simulink model "eBikeFinal"  (R2020b)
settings: Solver=daessc  StartTime=0.0  StopTime=60  FixedStep=1/500  AbsTol=1e-3  EnableMultiTasking=on
PreLoadFcn:
  | xh = 2*pi/60*[0:10:200];     % rpm to rad/s
  | yh = 50*(1-exp(-(max(xh)-xh)/2));
  | load bicycle_params
undefined symbols (not defined in the file or in its folder): sigbuilder_block
libraries: fl_lib x24, nesl_utility x15, sdl_lib x12, simulink x4, clutch_lib x3, motor_lib x3, LinearBrake_lib x2, pid_lib x2
settings Model: Creator=emcgarri  LastModifiedBy=amyyang
settings DataIOCC: SaveFormat=Array
settings OptimizationCC: BlockReduction=off  BufferReuse=off  LifeSpan=inf
settings DebuggingCC: ReadBeforeWriteMsg=DisableAll  WriteAfterWriteMsg=DisableAll  WriteAfterReadMsg=DisableAll  AlgebraicLoopMsg=none  UnderspecifiedInitializationDetection=Classic  MergeDetectMultiDrivingBlocksExec=none  MultiTaskDSMMsg=none  UnconnectedInputMsg=none  UnconnectedOutputMsg=none  UnconnectedLineMsg=none  SFUnexpectedBacktrackingDiag=warning  SFNoUnconditionalDefaultTransitionDiag=warning  SFExecutionAtInitializationDiag=none  ArithmeticOperatorsInVariantConditions=warning
settings HardwareCC: ProdBitPerPointer=32  ProdBitPerSizeT=32  ProdBitPerPtrDiffT=32  ProdLargestAtomicFloat=None  ProdIntDivRoundTo=Undefined  ProdEndianess=Unspecified  ProdWordSize=32  ProdHWDeviceType=32-bit Generic
settings ModelReferenceCC: UpdateModelReferenceTargets=IfOutOfDate  PropagateSignalLabelsOutOfModel=off
settings SFSimCC: SFSimEcho=off  SimUseLocalCustomCode=off
settings RTWCC: RTWUseLocalCustomCode=off
settings CodeAppCC: StateflowObjectComments=on
settings GRTTargetCC: TargetLangStandard=C89/C90 (ANSI)
settings ConfigComp: CovMetricSettings=dw  CovSaveCumulativeToWorkspaceVar=on  CovSaveSingleToWorkspaceVar=on  CovExternalEMLEnable=off  CovSFcnEnable=off
settings SimscapeCC: SimscapeNormalizeSystem=off

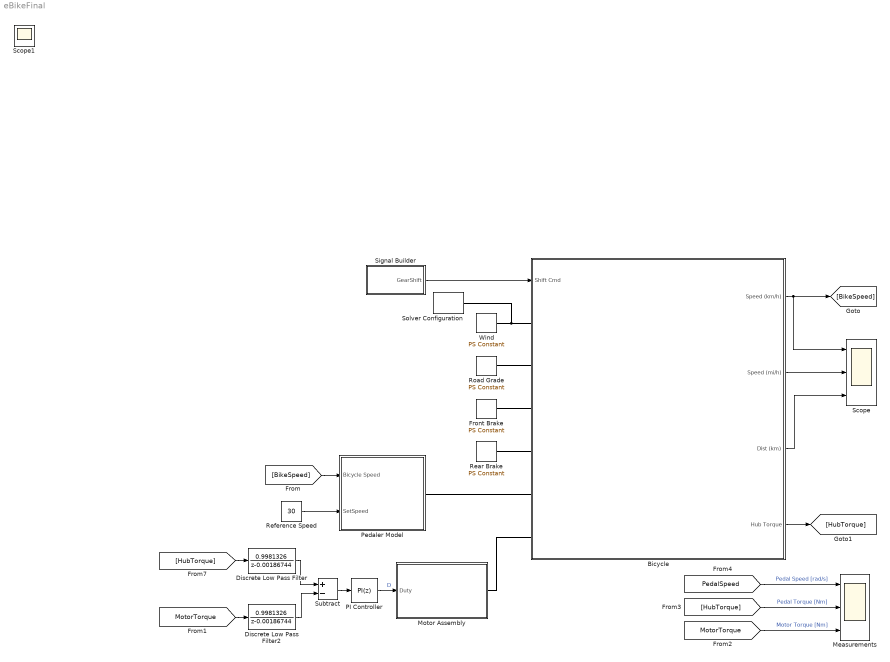
== system eBikeFinal ==
  Bicycle : Subsystem
      mask Display:
      | image(imread('FullBike.png'));
      | color('Orange')
      | port_label('input', 1, 'Gear');
      | port_label('lconn', 1, 'W');
      | port_label('lconn', 2, 'T');
      | port_label('lconn', 3, 'FB');
      | port_label('lconn', 4, 'RB');
      | port_label('lconn', 5, 'C');
      | port_label('lconn', 6, 'FH');
      | port_label('output', 1, 'Spd1');
      | port_label('output', 2, 'Spd2');
      | port_label('output', 3, 'Dist');
      | port_label('output', 4, 'TH');
  Discrete Low Pass Filter : DiscreteTransferFcn  Numerator=[0.9981326]  Denominator=[1 -0.00186744]  SampleTime=0.05
  Discrete Low Pass Filter2 : DiscreteTransferFcn  Numerator=[0.9981326]  Denominator=[1 -0.00186744]  SampleTime=0.05
  Front Brake : fl_lib/Physical Signals/Sources/PS Constant  constant=0 N
  Measurements : Scope  NumInputPorts=3
  Motor Assembly : Subsystem
      mask Display:
      | image(imread('MotorAssembly.png'));
      | color('Red');
      | port_label('input', 1, 'Duty');
      | port_label('rconn', 1, 'T');
  PI Controller : pid_lib/PID Controller  Controller=PI  Form=Parallel  TimeDomain=Discrete-time  UseExternalTs=off  SampleTime=0.05  IntegratorMethod=Forward Euler  FilterMethod=Forward Euler  ControllerParametersSource=internal  P=0.005  I=0.01  D=0.05  UseFilter=on  N=100  TunerSelectOption=Transfer Function Based (PID Tuner App)  InitialConditionSource=internal  InitialConditionForIntegrator=0  InitialConditionForFilter=0  DifferentiatorICPrevScaledInput=0  ExternalReset=none  IgnoreLimit=on  TrackingMode=off  Kt=1  LimitOutput=on  SatLimitsSource=internal  UpperSaturationLimit=1  LowerSaturationLimit=0  LinearizeAsGain=off  AntiWindupMode=clamping  Kb=1  POutMin=[]  POutMax=[]  IOutMin=[]  IOutMax=[]  DOutMin=[]  DOutMax=[]  NOutMin=[]  NOutMax=[]  SumOutMin=[]  SumOutMax=[]  SaturationOutMin=[]  SaturationOutMax=[]  PParamMin=[]  PParamMax=[]  IParamMin=[]  IParamMax=[]  DParamMin=[]  DParamMax=[]  NParamMin=[]  NParamMax=[]  KbParamMin=[]  KbParamMax=[]  KtParamMin=[]  KtParamMax=[]  KbOutMin=[]  KbOutMax=[]  KtOutMin=[]  KtOutMax=[]  IntegratorOutMin=[]  IntegratorOutMax=[]  FilterOutMin=[]  FilterOutMax=[]  SumI1OutMin=[]  SumI1OutMax=[]  SumI2OutMin=[]  SumI2OutMax=[]  SumI3OutMin=[]  SumI3OutMax=[]  SumI4OutMin=[]  SumI4OutMax=[]  SumDOutMin=[]  SumDOutMax=[]  DifferentiatorOutMin=[]  DifferentiatorOutMax=[]  FilterDiffOutCoefMin=[]  FilterDiffOutCoefMax=[]  ReciprocalOutMin=[]  ReciprocalOutMax=[]  SumDenOutMin=[]  SumDenOutMax=[]  SumNumOutMin=[]  SumNumOutMax=[]  DivideOutMin=[]  DivideOutMax=[]  UdiffTsProdOutMin=[]  UdiffTsProdOutMax=[]  NTsProdOutMin=[]  NTsProdOutMax=[]  UintegralTsProdOutMin=[]  UintegralTsProdOutMax=[]  UngainTsProdOutMin=[]  UngainTsProdOutMax=[]  IntegratorContinuousStateAttributes=''  IntegratorStateMustResolveToSignalObject=off  IntegratorRTWStateStorageClass=Auto  FilterContinuousStateAttributes=''  FilterStateMustResolveToSignalObject=off  FilterRTWStateStorageClass=Auto  ParallelPVariant=InternalParameters  IdealPVariant=Disabled  IVariant=InternalParameters  DVariant=Disabled  IntegratorVariant=Discrete  SatVariant=Enabled  AWVariant=DiscClampingParallel  PCopyVariant=Disabled  TRVariant=Disabled  FdbkBlocksVariant=Forward  IdealPFdbkVariant=Disabled  SatFdbkVariant=Disabled  DerivativeFilterVariant=Disabled  NVariant=Disabled  NCopyVariant=Disabled_SignalSpec  FilterICVariant=Disabled  IntegratorICVariant=InternalICs  ExternalResetVariant=Disabled  TRSumVariant=Passthrough  SumFdbkVariant=Disabled  SumVariant=Sum_PI  TsampFilterVariant=InternalTs  TsampNgainVariant=Passthrough  TsampIntegralVariant=Passthrough  ExternalSaturationOutDataTypeStr=Inherit: Same as second input
  Pedaler Model : Subsystem
      mask Display: image(imread('RiderIcon.png'));
  Rear Brake : fl_lib/Physical Signals/Sources/PS Constant  constant=0 N
  Reference Speed : Constant  Value=30
  Road Grade : fl_lib/Physical Signals/Sources/PS Constant  constant=0 deg
  Scope : Scope  NumInputPorts=3
  Signal Builder : Subsystem  Tag=STV Subsys  LoadFcn=sigbuilder_block('load');  StartFcn=sigbuilder_block('start');  StopFcn=sigbuilder_block('stop');  ClipboardFcn=sigbuilder_block('clipboard');  mask(Sigbuilder block){tuvar=[0:10]}
      mask help: Simulink:masks:SigbuilderBlock_MD
      mask init:
      | if ~strcmp(get_param(bdroot(gcbh),'SimulationStatus'),'stopped') tuvar = sigbuilder_block('maskInit'); end
      settings: CopyFcn=sigbuilder_block('copy');  DeleteFcn=sigbuilder_block('delete');  ModelCloseFcn=sigbuilder_block('modelClose');  PreSaveFcn=sigbuilder_block('preSave');  PauseFcn=sigbuilder_block('pause');  ContinueFcn=sigbuilder_block('continue');  NameChangeFcn=sigbuilder_block('namechange');  OpenFcn=sigbuilder_block('open',[306 225.6 549.6 399.6 ]);  CloseFcn=sigbuilder_block('close');
      mask Display: plot(0, 0, 100, 100,[2, 2, 32, 32, 2], [68, 8, 8, 68, 68],[32, 2], [38, 38], [32, 19, 2],[53, 60, 44], [32, 17, 17, 2],[16, 16, 31, 31]);txt = getActiveGroup(gcbh);text(2, 100, txt,'verticalAlignment', 'top');
  Solver Configuration : nesl_utility/Solver Configuration  PhysicalDomain=network_engine_domain  SubClassName=solver  LeftPortType=input  RightPortType=generic  Tones=[]  Harmonics=[]  SimulateNoise=off  Profile=off  UseLocalSampling=off  EnableSwitchedLinearOptims=on  FrequencyDomain=off  UseCCode=off  RelTol=0.001  AbsTol=1e-06  MinStep=1e-09  ToWorkspace=off  RevertToSquareIcSolve=off  NumHomotopyIterations=100  PhasorMode=off  PhasorModeNumHarmonics=1  DoDC=off  ResidualTolerance=1e-09  UseLocalSolver=off  LocalSolverChoice=NE_BACKWARD_EULER_ADVANCER  LocalSolverSampleTime=1e-3  DoFixedCost=off  MaxNonlinIter=3  MaxModeIter=2  ComputeImpulses=off  ImpulseIterations=1  LinearAlgebra=Sparse  EquationFormulation=NE_TIME_EF  DelaysMemoryBudget=1024  AutomaticFiltering=off  FilteringTimeConstant=0.001  PartitionStorageMethod=AS_NEEDED  PartitionMemoryBudget=1024  PartitionMethod=FAST
  Subtract : Sum  Inputs=+-
  Wind : fl_lib/Physical Signals/Sources/PS Constant  constant=0 m/s
  Scope1 : Scope
  wires:
  [BikeSpeed] -> Pedaler Model/1(Bicycle Speed)
  Reference Speed/1 -> Pedaler Model/2(SetSpeed)
  [HubTorque] -> Measurements/2  "Pedal Torque [Nm]"
  [MotorTorque] -> Measurements/3  "Motor Torque [Nm]"
  [PedalSpeed] -> Measurements/1  "Pedal Speed [rad/s]"
  Signal Builder/1(GearShift) -> Bicycle/1(Shift Cmd)
  PI Controller/1 -> Motor Assembly/1(Duty)  "D"
  [MotorTorque] -> Discrete Low Pass Filter2/1
  Subtract/1 -> PI Controller/1
  [HubTorque] -> Discrete Low Pass Filter/1
  Discrete Low Pass Filter2/1 -> Subtract/2
  Discrete Low Pass Filter/1 -> Subtract/1
  Bicycle/2(Speed (mi/h)) -> Scope/2
  Bicycle/3(Dist (km)) -> Scope/3
  Bicycle/4(Hub Torque) -> [HubTorque]
  Bicycle/1(Speed (km/h)) -> Scope/1, [BikeSpeed]
  connections:
  Bicycle/LConn5 -- Pedaler Model/RConn1
  Bicycle/LConn3 -- Front Brake/RConn1
  Bicycle/LConn4 -- Rear Brake/RConn1
  Bicycle/LConn2 -- Road Grade/RConn1
  Wind/RConn1 -- Bicycle/LConn1 -- Solver Configuration/RConn1
  Bicycle/LConn6 -- Motor Assembly/RConn1

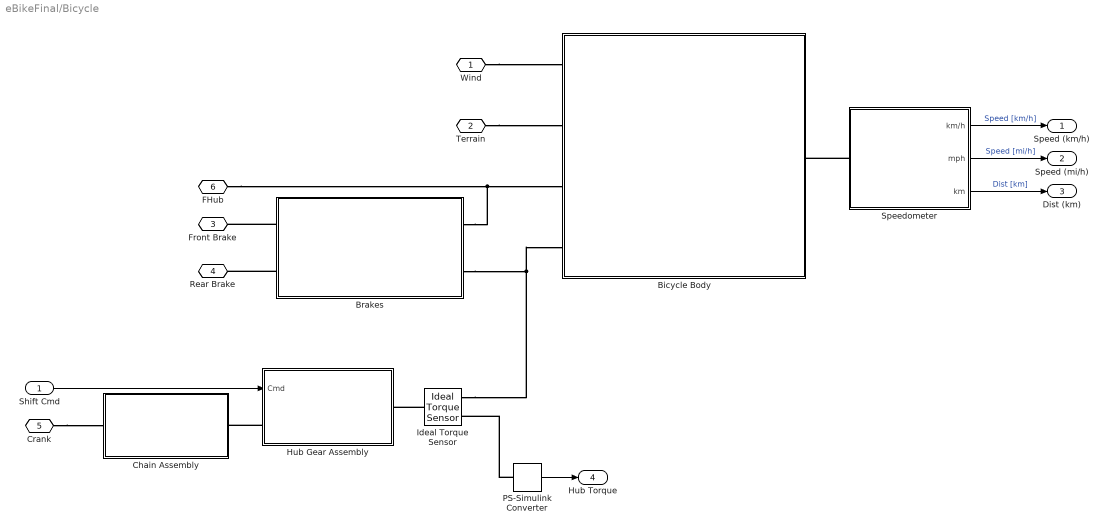
== system eBikeFinal/Bicycle ==
  Shift Cmd : Inport
  "Bicycle Body " : Subsystem  mask(Vehicle){rider_mass=80, rider_area=0.8, drag_coeff=0.5, bike_mass=13, front_axle=47, rear_axle=65, CG_height=120, rim_radius=311, tire_height=41, tire_friction_s=1.0, tire_friction_k=0.7, roll_resist=0.004}
      mask prompts: rider_mass "Mass [kg]"; rider_area "Area [m^2]"; drag_coeff "Drag Coefficient"; bike_mass "Frame Mass [kg]"; front_axle "Front Axle Loc [cm]"; rear_axle "Real Axle Loc [cm]"; CG_height "CG Height [cm]"; rim_radius "Rim Radius [mm]"; tire_height "Tire Height [mm]"; tire_friction_s "Static Tire Friction"; tire_friction_k "Kinetic Tire Friction"; roll_resist "Rolling Resistance"
      mask help:
      | This block represents a simple bicycle body with drive attachments on both
      | the front and rear hubs.
      mask Display:
      | image(imread('BikeIcon.png'));
      | color('Orange')
      | port_label('lconn', 1, 'W');
      | port_label('lconn', 2, 'T');
      | port_label('rconn', 1, 'H');
      | port_label('lconn', 3, 'F');
      | port_label('lconn', 4, 'R');
  Brakes : Subsystem
      mask Display:
      | image(imread('HandleBars.png'));
      | color('Red');
      | port_label('lconn', 1, 'FCmd');
      | port_label('lconn', 2, 'RCmd');
      | port_label('rconn', 1, 'FB');
      | port_label('rconn', 2, 'RB');
  Chain Assembly : Subsystem
      mask Display:
      | image(imread('ChainDrive.png'))
      | color('Orange')
      | port_label('lconn', 1, 'C');
      | port_label('rconn', 1, 'H');
  Hub Gear Assembly : Subsystem
      mask Display:
      | image(imread('HubTrans.png'))
      | color('Orange')
      | port_label('input', 1, 'Cmd');
      | port_label('lconn', 1, 'A');
      | port_label('rconn', 1, 'H');
  Ideal Torque Sensor : fl_lib/Mechanical/Mechanical Sensors/Ideal Torque Sensor
  PS-Simulink Converter : nesl_utility/PS-Simulink Converter  PhysicalDomain=network_engine_domain  SubClassName=ps_output  LeftPortType=input  RightPortType=output  PseudoPeriodic=off  Frequencies=[]  Unit=N*m  AffineConversion=off
  Speedometer : Subsystem  mask(Speedometer){}
      mask help:
      | Simple speedometer/odometer. The input signal should be a physical signal
      | with units of m/s. The output signals are km/h, mi/h and km traveled as
      | Simulink signals for convenient plotting.
      mask Display:
      | image(imread('SpeedometerIcon.png'));
      | color('Orange')
      | port_label('lconn', 1, 'H');
      | port_label('output', 1, 'km/h');
      | port_label('output', 2, 'mi/h');
      | port_label('output', 3, 'km');
  Wind : PMIOPort  Side=Left
  Terrain : PMIOPort  Port=2  Side=Left
  Front Brake : PMIOPort  Port=3  Side=Left
  Rear Brake : PMIOPort  Port=4  Side=Left
  Crank : PMIOPort  Port=5  Side=Left
  FHub : PMIOPort  Port=6  Side=Left
  Speed (km/h) : Outport  VectorParamsAs1DForOutWhenUnconnected=off
  Speed (mi/h) : Outport  Port=2  VectorParamsAs1DForOutWhenUnconnected=off
  Dist (km) : Outport  Port=3  VectorParamsAs1DForOutWhenUnconnected=off
  Hub Torque : Outport  Port=4  VectorParamsAs1DForOutWhenUnconnected=off
  wires:
  Speedometer/1(km/h) -> Speed (km/h)/1  "Speed [km/h]"
  Speedometer/2(mph) -> Speed (mi/h)/1  "Speed [mi/h]"
  Speedometer/3(km) -> Dist (km)/1  "Dist [km]"
  Shift Cmd/1 -> Hub Gear Assembly/1(Cmd)
  PS-Simulink Converter/1 -> Hub Torque/1
  connections:
  Wind/RConn1 -- "Bicycle Body "/LConn1
  Terrain/RConn1 -- "Bicycle Body "/LConn2
  Speedometer/LConn1 -- "Bicycle Body "/RConn1
  Brakes/LConn1 -- Front Brake/RConn1
  Brakes/LConn2 -- Rear Brake/RConn1
  Hub Gear Assembly/LConn1 -- Chain Assembly/RConn1
  FHub/RConn1 -- Brakes/RConn1 -- "Bicycle Body "/LConn3
  Brakes/RConn2 -- "Bicycle Body "/LConn4 -- Ideal Torque Sensor/RConn1
  Crank/RConn1 -- Chain Assembly/LConn1
  PS-Simulink Converter/LConn1 -- Ideal Torque Sensor/RConn2
  Ideal Torque Sensor/LConn1 -- Hub Gear Assembly/RConn1

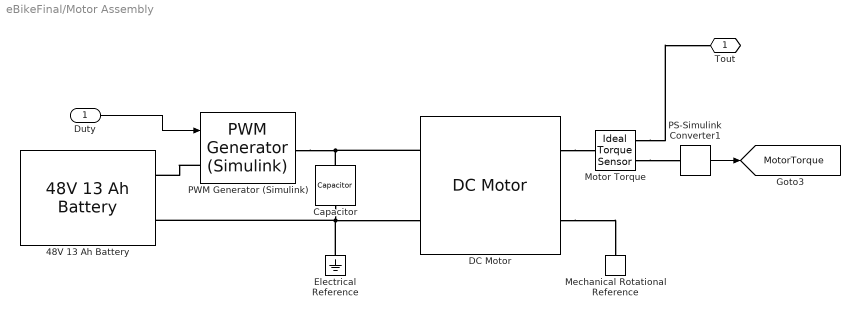
== system eBikeFinal/Motor Assembly ==
  Duty : Inport
  48V 13 Ah Battery : motor_lib/48V 13 Ah Battery  SystemSampleTime=-1  VariantActivationTime=update diagram  Latency=0  AutoFrameSizeCalculation=off
  Capacitor : fl_lib/Electrical/Electrical Elements/Capacitor  c=0.2 F  r=1e-6 Ohm  g=0 1/Ohm  i_specify=off  i_priority=None  i=0 A  i_nominal_specify=off  i_nominal_unit=A  i_nominal_value=1  v_specify=off  v_priority=None  v=0 V  v_nominal_specify=off  v_nominal_unit=V  v_nominal_value=1  vc_specify=on  vc_priority=High  vc=0 V  vc_nominal_specify=off  vc_nominal_unit=V  vc_nominal_value=1
  DC Motor : motor_lib/DC Motor  SystemSampleTime=-1  VariantActivationTime=update diagram  Latency=0  AutoFrameSizeCalculation=off
  Electrical Reference : fl_lib/Electrical/Electrical Elements/Electrical Reference
  Mechanical Rotational Reference : fl_lib/Mechanical/Rotational Elements/Mechanical Rotational Reference
  Motor Torque : fl_lib/Mechanical/Mechanical Sensors/Ideal Torque Sensor
  PS-Simulink Converter1 : nesl_utility/PS-Simulink Converter  PhysicalDomain=network_engine_domain  SubClassName=ps_output  LeftPortType=input  RightPortType=output  PseudoPeriodic=off  Frequencies=[]  Unit=1  AffineConversion=off
  PWM Generator (Simulink) : motor_lib/PWM Generator  (Simulink)  freq=50  Ts=2e-4
  Tout : PMIOPort  Side=Right
  tag scope: MotorTorque=global
  wires:
  PS-Simulink Converter1/1 -> [MotorTorque]
  Duty/1 -> PWM Generator (Simulink)/1
  connections:
  DC Motor/RConn2 -- Mechanical Rotational Reference/LConn1
  DC Motor/LConn1 -- PWM Generator (Simulink)/RConn1 -- Capacitor/LConn1
  PWM Generator (Simulink)/LConn1 -- 48V 13 Ah Battery/RConn1
  DC Motor/RConn1 -- Motor Torque/LConn1
  Motor Torque/RConn2 -- PS-Simulink Converter1/LConn1
  Motor Torque/RConn1 -- Tout/RConn1
  Capacitor/RConn1 -- Electrical Reference/LConn1 -- 48V 13 Ah Battery/RConn2 -- DC Motor/LConn2

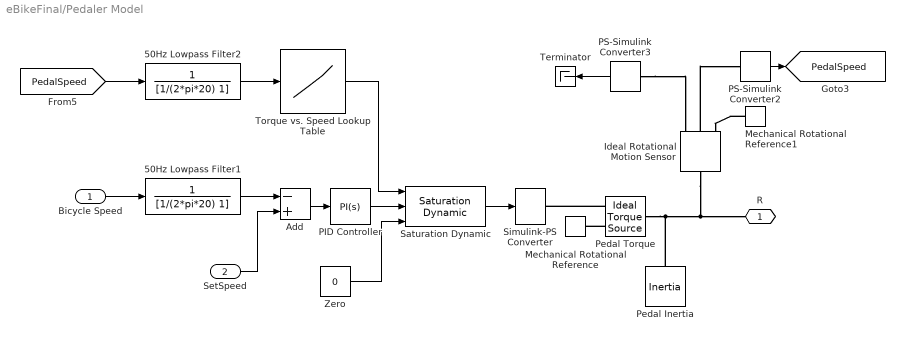
== system eBikeFinal/Pedaler Model ==
  Bicycle Speed : Inport
  SetSpeed : Inport  Port=2
  50Hz Lowpass Filter1 : TransferFcn  Denominator=[1/(2*pi*20) 1]
  50Hz Lowpass Filter2 : TransferFcn  Denominator=[1/(2*pi*20) 1]
  Add : Sum  Inputs=-+
  Ideal Rotational Motion Sensor : fl_lib/Mechanical/Mechanical Sensors/Ideal Rotational Motion Sensor  wrap_angle=simscape.enum.onoff.off  offset=0 rad
  Mechanical Rotational Reference : fl_lib/Mechanical/Rotational Elements/Mechanical Rotational Reference
  Mechanical Rotational Reference1 : fl_lib/Mechanical/Rotational Elements/Mechanical Rotational Reference
  PID Controller : pid_lib/PID Controller  Controller=PI  Form=Parallel  TimeDomain=Continuous-time  UseExternalTs=off  SampleTime=-1  IntegratorMethod=Forward Euler  FilterMethod=Forward Euler  ControllerParametersSource=internal  P=20  I=0  D=0  UseFilter=on  N=100  TunerSelectOption=Transfer Function Based (PID Tuner App)  InitialConditionSource=internal  InitialConditionForIntegrator=0  InitialConditionForFilter=0  DifferentiatorICPrevScaledInput=0  ExternalReset=none  TrackingMode=off  Kt=1  LimitOutput=off  SatLimitsSource=internal  UpperSaturationLimit=50  LowerSaturationLimit=0  LinearizeAsGain=on  AntiWindupMode=clamping  Kb=1  POutMin=[]  POutMax=[]  IOutMin=[]  IOutMax=[]  DOutMin=[]  DOutMax=[]  NOutMin=[]  NOutMax=[]  SumOutMin=[]  SumOutMax=[]  SaturationOutMin=[]  SaturationOutMax=[]  PParamMin=[]  PParamMax=[]  IParamMin=[]  IParamMax=[]  DParamMin=[]  DParamMax=[]  NParamMin=[]  NParamMax=[]  KbParamMin=[]  KbParamMax=[]  KtParamMin=[]  KtParamMax=[]  KbOutMin=[]  KbOutMax=[]  KtOutMin=[]  KtOutMax=[]  IntegratorOutMin=[]  IntegratorOutMax=[]  FilterOutMin=[]  FilterOutMax=[]  SumI1OutMin=[]  SumI1OutMax=[]  SumI2OutMin=[]  SumI2OutMax=[]  SumI3OutMin=[]  SumI3OutMax=[]  SumI4OutMin=[]  SumI4OutMax=[]  SumDOutMin=[]  SumDOutMax=[]  DifferentiatorOutMin=[]  DifferentiatorOutMax=[]  FilterDiffOutCoefMin=[]  FilterDiffOutCoefMax=[]  ReciprocalOutMin=[]  ReciprocalOutMax=[]  SumDenOutMin=[]  SumDenOutMax=[]  SumNumOutMin=[]  SumNumOutMax=[]  DivideOutMin=[]  DivideOutMax=[]  UdiffTsProdOutMin=[]  UdiffTsProdOutMax=[]  NTsProdOutMin=[]  NTsProdOutMax=[]  UintegralTsProdOutMin=[]  UintegralTsProdOutMax=[]  UngainTsProdOutMin=[]  UngainTsProdOutMax=[]  IntegratorContinuousStateAttributes=''  IntegratorStateMustResolveToSignalObject=off  IntegratorRTWStateStorageClass=Auto  FilterContinuousStateAttributes=''  FilterStateMustResolveToSignalObject=off  FilterRTWStateStorageClass=Auto  ParallelPVariant=InternalParameters  IdealPVariant=Disabled  IVariant=InternalParameters  DVariant=Disabled  IntegratorVariant=Continuous  SatVariant=Disabled  AWVariant=Passthrough  PCopyVariant=Disabled  TRVariant=Disabled  FdbkBlocksVariant=Forward  IdealPFdbkVariant=Disabled  SatFdbkVariant=Disabled  DerivativeFilterVariant=Disabled  NVariant=Disabled  NCopyVariant=Disabled_SignalSpec  FilterICVariant=Disabled  IntegratorICVariant=InternalICs  ExternalResetVariant=Disabled  TRSumVariant=Passthrough  SumFdbkVariant=Disabled  SumVariant=Sum_PI  TsampFilterVariant=InternalTs  TsampNgainVariant=Passthrough  TsampIntegralVariant=Passthrough  ExternalSaturationOutDataTypeStr=Inherit: Same as second input
  PS-Simulink Converter2 : nesl_utility/PS-Simulink Converter  PhysicalDomain=network_engine_domain  SubClassName=ps_output  LeftPortType=input  RightPortType=output  PseudoPeriodic=off  Frequencies=[]  Unit=rad/s  AffineConversion=off
  PS-Simulink Converter3 : nesl_utility/PS-Simulink Converter  PhysicalDomain=network_engine_domain  SubClassName=ps_output  LeftPortType=input  RightPortType=output  PseudoPeriodic=off  Frequencies=[]  Unit=1  AffineConversion=off
  Pedal Inertia : fl_lib/Mechanical/Rotational Elements/Inertia  inertia=0.025 kg*m^2  num_ports=foundation.enum.numPorts2.one  w_specify=off  w_priority=High  w=0 rad/s  w_nominal_specify=off  w_nominal_unit=rad/s  w_nominal_value=1  t_specify=off  t_priority=High  t=0 N*m  t_nominal_specify=off  t_nominal_unit=N*m  t_nominal_value=1
  Pedal Torque : fl_lib/Mechanical/Mechanical Sources/Ideal Torque Source
  Saturation Dynamic : simulink/Discontinuities/Saturation Dynamic  OutMin=[]  OutMax=[]  OutDataTypeStr=Inherit: Same as second input  OutDataType=fixdt(1, 16)  OutScaling=2^-10  DoSatur=off
  Simulink-PS Converter : nesl_utility/Simulink-PS Converter  PhysicalDomain=network_engine_domain  SubClassName=ps_input  LeftPortType=input  RightPortType=output  PseudoPeriodic=off  Frequencies=[]  NoiseDistribution=none  NoiseParameters=[]  Unit=N*m  AffineConversion=off  FilteringAndDerivatives=filter  SimscapeFilterOrder=1  InputFilterTimeConstant=0.001  UdotUserProvided=1
  Terminator : Terminator
  Torque vs. Speed Lookup Table : Lookup_n-D  NumberOfTableDimensions=1  BreakpointsForDimension1=xh  Table=yh  ExtrapMethod=Clip  RndMeth=Simplest  InputSameDT=on
  Zero : Constant  Value=0
  R : PMIOPort  Side=Right
  tag scope: PedalSpeed=global
  wires:
  SetSpeed/1 -> Add/2
  Add/1 -> PID Controller/1
  Zero/1 -> Saturation Dynamic/3
  Bicycle Speed/1 -> 50Hz Lowpass Filter1/1
  50Hz Lowpass Filter2/1 -> Torque vs. Speed Lookup Table/1
  50Hz Lowpass Filter1/1 -> Add/1
  Torque vs. Speed Lookup Table/1 -> Saturation Dynamic/1
  PID Controller/1 -> Saturation Dynamic/2
  Saturation Dynamic/1 -> Simulink-PS Converter/1
  [PedalSpeed] -> 50Hz Lowpass Filter2/1
  PS-Simulink Converter2/1 -> [PedalSpeed]
  PS-Simulink Converter3/1 -> Terminator/1
  connections:
  Pedal Torque/LConn1 -- Ideal Rotational Motion Sensor/LConn1 -- R/RConn1 -- Pedal Inertia/LConn1
  Pedal Torque/RConn2 -- Mechanical Rotational Reference/LConn1
  Pedal Torque/RConn1 -- Simulink-PS Converter/RConn1
  Ideal Rotational Motion Sensor/RConn2 -- PS-Simulink Converter2/LConn1
  PS-Simulink Converter3/LConn1 -- Ideal Rotational Motion Sensor/RConn3
  Mechanical Rotational Reference1/LConn1 -- Ideal Rotational Motion Sensor/RConn1

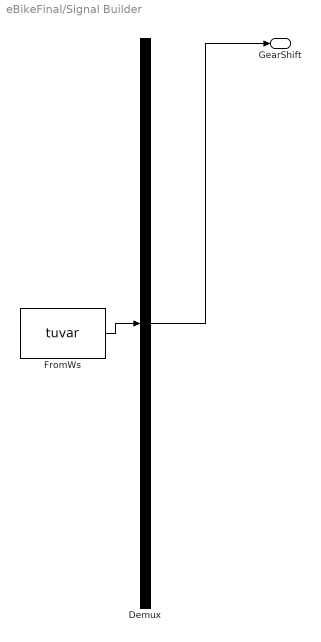
== system eBikeFinal/Signal Builder ==
  Demux : Demux  Tag=STV Demux  Outputs=1
      settings: DisplayOption=none
  FromWs : FromWorkspace  Tag=STV FromWs  VariableName=tuvar
      SigBuilderData=|
      | common.afterFinalStr = 'Extrapolate'
      | common.sampleTime = 0
      | dataSet.timeRange = [0 60]
      | dataSet.name = 'Gear'
      | sbobj.Groups.Name = 'Gear'
      | sbobj.Groups.Signals.Name = 'GearShift'
      | sbobj.Groups.Signals.XData = [0 5 5 35 35 60]
      | sbobj.Groups.Signals.YData = [1 1 2 2 3 3]
      | sbobj.Groups.TimeRange = [0 60]
  GearShift : Outport  Tag=STV Outport  VectorParamsAs1DForOutWhenUnconnected=off
  wires:
  Demux/1 -> GearShift/1
  FromWs/1 -> Demux/1

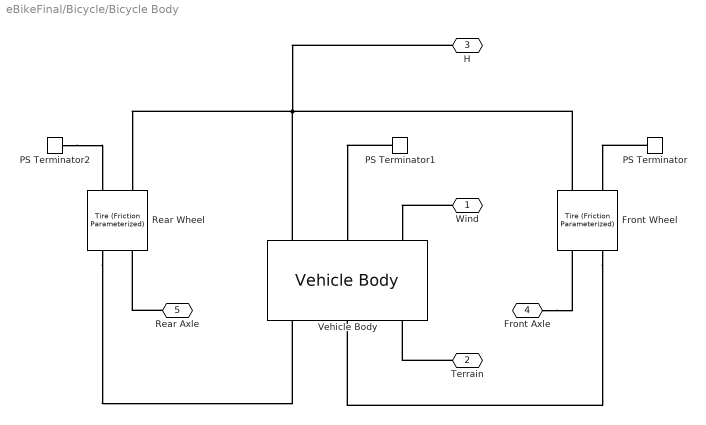
== system eBikeFinal/Bicycle/Bicycle Body  ==
  Front Wheel : sdl_lib/Tires & Vehicles/Tire (Friction Parameterized)  r_tire=rim_radius + tire_height mm  friction_model=1  mu_static=tire_friction_s  mu_kinetic=tire_friction_k  slip_vector=[ 0 0.02 0.06 0.15 0.6 1 ] rad/s  mu_kinetic_vector=[ 0.89 0.88 0.8 0.75 0.7 0.7 ]  interp_method=1  extrap_method=1  model_compliance=0  stiffness=1e+6 N/m  damping=1000 N/(m/s)  model_inertia=1  tire_inertia=tire_inertia kg*m^2  initial_velocity=0 rad/s  model_resistance=1  resistance_model=1  coeff=roll_resist  p_tire=250e3 Pa  alpha=-0.003  beta=0.97  coeff_a=84e-4  coeff_b=6.2e-4 s/m  coeff_c=1.6e-4 s^2/m^2  v_thr=1e-3 m/s  v_tol=0.01 m/s  F_min=10 N  initial_traction_state=1
      settings: SourceProductBaseCode=LD  InternalSimscapePortConfiguration="{\"Bottom\":[],\"Left\":[{\"id\":\"N\",\"label\":\"N\",\"type\":\"input\"},{\"id\":\"A\",\"label\":\"A\",\"type\":\"foundation.mechanical.rotational.rotational\"}],\"Right\":[{\"id\":\"S\",\"label\":\"S\",\"type\":\"output\"},{\"id\":\"H\",\"label\":\"H\",\"type\":\"foundation.mechanical.translational.translational\"}],\"Top\":[]}"
  PS Terminator : fl_lib/Physical Signals/Sinks/PS Terminator
  PS Terminator1 : fl_lib/Physical Signals/Sinks/PS Terminator
  PS Terminator2 : fl_lib/Physical Signals/Sinks/PS Terminator
  Rear Wheel : sdl_lib/Tires & Vehicles/Tire (Friction Parameterized)  r_tire=rim_radius + tire_height mm  friction_model=1  mu_static=tire_friction_s  mu_kinetic=tire_friction_k  slip_vector=[ 0 0.02 0.06 0.15 0.6 1 ] rad/s  mu_kinetic_vector=[ 0.89 0.88 0.8 0.75 0.7 0.7 ]  interp_method=1  extrap_method=1  model_compliance=0  stiffness=1e+6 N/m  damping=1000 N/(m/s)  model_inertia=1  tire_inertia=tire_inertia kg*m^2  initial_velocity=0 rad/s  model_resistance=1  resistance_model=1  coeff=roll_resist  p_tire=250e3 Pa  alpha=-0.003  beta=0.97  coeff_a=84e-4  coeff_b=6.2e-4 s/m  coeff_c=1.6e-4 s^2/m^2  v_thr=1e-3 m/s  v_tol=0.01 m/s  F_min=10 N  initial_traction_state=1
      settings: SourceProductBaseCode=LD  InternalSimscapePortConfiguration="{\"Bottom\":[],\"Left\":[{\"id\":\"N\",\"label\":\"N\",\"type\":\"input\"},{\"id\":\"A\",\"label\":\"A\",\"type\":\"foundation.mechanical.rotational.rotational\"}],\"Right\":[{\"id\":\"S\",\"label\":\"S\",\"type\":\"output\"},{\"id\":\"H\",\"label\":\"H\",\"type\":\"foundation.mechanical.translational.translational\"}],\"Top\":[]}"
  Vehicle Body : sdl_lib/Tires & Vehicles/Vehicle Body  mass=rider_mass + bike_mass kg  n_w=1  x_f=front_axle cm  x_r=rear_axle cm  y_c=CG_height cm  mass_var=simscape.enum.onoff.off  model_pitch=0  inertia=4000 kg*m^2  suspension_model=1  k_f=1e4 N/m  b_f=1e4 N/(m/s)  k_r=1e4 N/m  b_r=1e4 N/(m/s)  k_f_TLU=[-2000, -1000, 0, 1000, 2000] N  x_f_TLU=[-.4, -.2, 0, .2, .4] m  b_f_TLU=[-200, -100, 0, 100, 200] N  v_f_TLU=[-4, -2, 0, 2, 4] m/s  k_r_TLU=[-2000, -1000, 0, 1000, 2000] N  x_r_TLU=[-.4, -.2, 0, .2, .4] m  b_r_TLU=[-200, -100, 0, 100, 200] N  v_r_TLU=[-4, -2, 0, 2, 4] m/s  interp_method=simscape.enum.interpolation.linear  extrap_method=simscape.enum.extrapolation.linear  model_hardstop=0  upper_bound_f=.25 m  lower_bound_f=-.25 m  stop_k_f=1e6 N/m  stop_b_f=150 N/(m/s)  upper_bound_r=.25 m  lower_bound_r=-.25 m  stop_k_r=1e6 N/m  stop_b_r=150 N/(m/s)  initial_pitch=0 rad  initial_pitch_rate=0 rad/s  g=9.81 m/s^2  liftoff_warning=0  area=rider_area m^2  Cd=drag_coeff  rho=1.18 kg/m^3  v_specify=on  v_priority=High  v=0 m/s  v_nominal_specify=off  v_nominal_unit=m/s  v_nominal_value=1
  Wind : PMIOPort  Side=Left
  Terrain : PMIOPort  Port=2  Side=Left
  H : PMIOPort  Port=3  Side=Right
  Front Axle : PMIOPort  Port=4  Side=Left
  Rear Axle : PMIOPort  Port=5  Side=Left
  connections:
  Front Wheel/RConn2 -- Vehicle Body/LConn1 -- H/RConn1 -- Rear Wheel/RConn2
  Front Wheel/LConn1 -- Vehicle Body/RConn2
  Front Axle/RConn1 -- Front Wheel/LConn2
  Terrain/RConn1 -- Vehicle Body/RConn3
  Rear Wheel/LConn1 -- Vehicle Body/RConn1
  PS Terminator2/LConn1 -- Rear Wheel/RConn1
  PS Terminator1/LConn1 -- Vehicle Body/LConn2
  Wind/RConn1 -- Vehicle Body/LConn3
  PS Terminator/LConn1 -- Front Wheel/RConn1
  Rear Axle/RConn1 -- Rear Wheel/LConn2

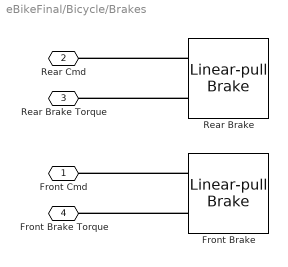
== system eBikeFinal/Bicycle/Brakes ==
  Front Brake : LinearBrake_lib/Linear-pull Brake  r_rim=311 mm  r_c=100 mm  r_b=40 mm  mu=0.7  mu_visc=0.35 N*m/(rad/s)  w_thr=0.01 rad/s  w_rim_specify=off  w_rim_priority=High  w_rim=0 rad/s  w_rim_nominal_specify=off  w_rim_nominal_unit=rad/s  w_rim_nominal_value=1  t_rim_specify=off  t_rim_priority=High  t_rim=0 N*m  t_rim_nominal_specify=off  t_rim_nominal_unit=N*m  t_rim_nominal_value=1
      settings: InternalSimscapePortConfiguration="{\"Bottom\":[],\"Left\":[{\"id\":\"Fc\",\"label\":\"Fc\",\"type\":\"input\"},{\"id\":\"S\",\"label\":\"S\",\"type\":\"foundation.mechanical.rotational.rotational\"}],\"Right\":[],\"Top\":[]}"
  Rear Brake : LinearBrake_lib/Linear-pull Brake  r_rim=311 mm  r_c=100 mm  r_b=40 mm  mu=0.7  mu_visc=0.35 N*m/(rad/s)  w_thr=0.01 rad/s  w_rim_specify=off  w_rim_priority=High  w_rim=0 rad/s  w_rim_nominal_specify=off  w_rim_nominal_unit=rad/s  w_rim_nominal_value=1  t_rim_specify=off  t_rim_priority=High  t_rim=0 N*m  t_rim_nominal_specify=off  t_rim_nominal_unit=N*m  t_rim_nominal_value=1
      settings: InternalSimscapePortConfiguration="{\"Bottom\":[],\"Left\":[{\"id\":\"Fc\",\"label\":\"Fc\",\"type\":\"input\"},{\"id\":\"S\",\"label\":\"S\",\"type\":\"foundation.mechanical.rotational.rotational\"}],\"Right\":[],\"Top\":[]}"
  Front Cmd : PMIOPort  Side=Left
  Rear Cmd : PMIOPort  Port=2  Side=Left
  Rear Brake Torque : PMIOPort  Port=3  Side=Right
  Front Brake Torque : PMIOPort  Port=4  Side=Right
  connections:
  Front Brake/LConn1 -- Front Cmd/RConn1
  Rear Brake/LConn2 -- Rear Brake Torque/RConn1
  Rear Brake/LConn1 -- Rear Cmd/RConn1
  Front Brake/LConn2 -- Front Brake Torque/RConn1

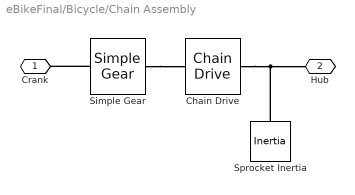
== system eBikeFinal/Bicycle/Chain Assembly ==
  Chain Drive : sdl_lib/Couplings & Drives/Chain Drive  chain_model=2  radius_a=12.7/(2*sin(pi/39)) mm  radius_b=12.7/(2*sin(pi/14)) mm  slack=6.35 mm  k_chain=1e6 N/m  mu_visc_chain=5e5 N/(m/s)  mu_visc_a=0.001 N*m/(rad/s)  mu_visc_b=0.001 N*m/(rad/s)  breakable=0  F_max=1e+6 N  x_specify=on  x_priority=High  x=0 mm  x_nominal_specify=off  x_nominal_unit=mm  x_nominal_value=1
      settings: SourceProductBaseCode=LD  InternalSimscapePortConfiguration="{\"Bottom\":[],\"Left\":[{\"id\":\"A\",\"label\":\"A\",\"type\":\"foundation.mechanical.rotational.rotational\"}],\"Right\":[{\"id\":\"B\",\"label\":\"B\",\"type\":\"foundation.mechanical.rotational.rotational\"}],\"Top\":[]}"
  Simple Gear : sdl_lib/Gears/Simple Gear  ratio=2  rotation_direction=3-2*(1)  friction_model=1  mu_visc=[ 0 0 ] N*m/(rad/s)  T_noload=0.1 N*m  T_nom=5 N*m  efficiency_nom=0.8  efficiency=0.8  temperature_TLU=[ 280 300 320 ] K  load_TLU=[ 1 5 10 ] N*m  efficiency_TLU=[ 0.95 0.9 0.85 ]  efficiency_TLU2=[ 0.85 0.8 0.75; 0.95 0.9 0.85; 0.85 0.8 0.7 ]  w_thr=0.01 rad/s  pwr_thr=0.001 W  thermal_mass=50 J/K  enable_faults=simscape.enum.onoff.off  efficiency_fault=0.05  external_fault=simscape.enum.onoff.off  temporal_fault=simscape.enum.onoff.off  fault_time=5 s  fault_angles=pi / 12 rad  report_fault=(1)-1  temperature_specify=off  temperature_priority=High  temperature=300 K  temperature_nominal_specify=off  temperature_nominal_unit=K  temperature_nominal_value=1
  Sprocket Inertia : fl_lib/Mechanical/Rotational Elements/Inertia  inertia=0.0005 kg*m^2  num_ports=foundation.enum.numPorts2.one  w_specify=on  w_priority=High  w=0 rad/s  w_nominal_specify=off  w_nominal_unit=rad/s  w_nominal_value=1  t_specify=off  t_priority=High  t=0 N*m  t_nominal_specify=off  t_nominal_unit=N*m  t_nominal_value=1
  Crank : PMIOPort  Side=Left
  Hub : PMIOPort  Port=2  Side=Right
  connections:
  Simple Gear/LConn1 -- Crank/RConn1
  Simple Gear/RConn1 -- Chain Drive/LConn1
  Chain Drive/RConn1 -- Hub/RConn1 -- Sprocket Inertia/LConn1

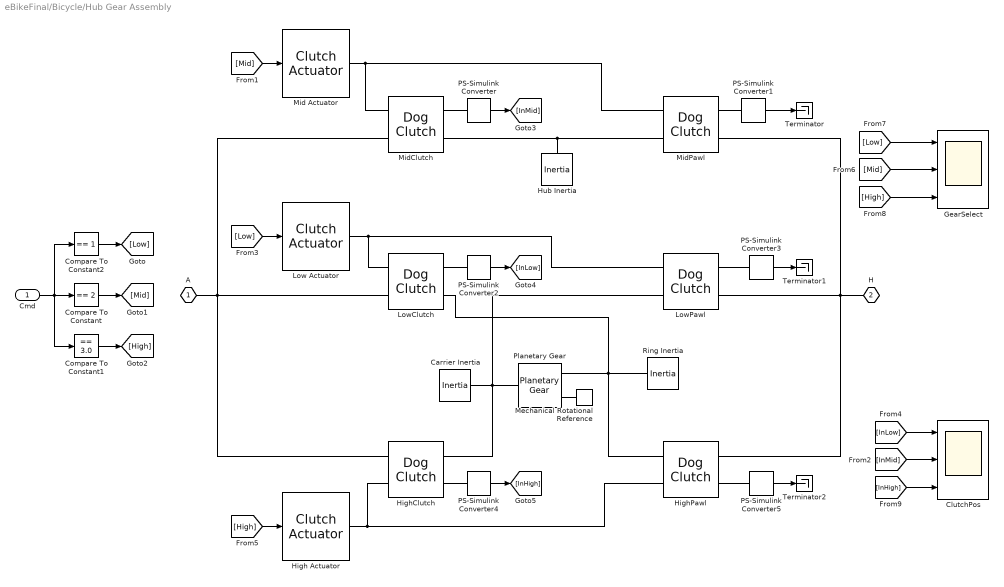
== system eBikeFinal/Bicycle/Hub Gear Assembly ==
  Cmd : Inport
  Carrier Inertia : fl_lib/Mechanical/Rotational Elements/Inertia  inertia=0.0005 kg*m^2  num_ports=foundation.enum.numPorts2.one  w_specify=on  w_priority=High  w=0 rad/s  w_nominal_specify=off  w_nominal_unit=rad/s  w_nominal_value=1  t_specify=off  t_priority=High  t=0 N*m  t_nominal_specify=off  t_nominal_unit=N*m  t_nominal_value=1
  ClutchPos : Scope  NumInputPorts=3
  Compare To Constant : simulink/Logic and Bit Operations/Compare To Constant  relop===  const=2  OutDataTypeStr=boolean
  Compare To Constant1 : simulink/Logic and Bit Operations/Compare To Constant  relop===  const=3.0  OutDataTypeStr=boolean
  Compare To Constant2 : simulink/Logic and Bit Operations/Compare To Constant  relop===  const=1  OutDataTypeStr=boolean
  GearSelect : Scope  NumInputPorts=3
  High Actuator : clutch_lib/Clutch Actuator  SystemSampleTime=-1  VariantActivationTime=update diagram  Latency=0  AutoFrameSizeCalculation=off
  HighClutch : sdl_lib/Clutches/Dog Clutch  thermal_port=simscape.enum.thermaleffects.omit  model=1  max_torque=1000 N*m  temperature_TLU=[280.0, 300.0, 320.0] K  max_torque_vector=[1000.0, 1050.0, 1000.0] N*m  interp_method=1  extrap_method=1  radius=10 mm  n_teeth=6  clutch_backlash=10 deg  clutch_stiffness=1e+7 N*m/rad  clutch_damping=100 N*m/(rad/s)  shift_linkage=sdl.enum.shift_linkage.conserving  tooth_height=3 mm  ring_hub_gap=1 mm  back_stop=1  transl_stiffness=1e+6 N/m  transl_damping=1000 N/(m/s)  visc_fric_transl=100 N/(m/s)  fric_coeff=0.05  direction=3-2*(1)  engagement_velocity=inf rpm  engagement_overlap=1 mm  initial_state_engaged=0  init_pos=0 mm  init_rel_angle=0 deg  thermal_mass=25 kJ/K  T_init=300 K
      settings: SourceProductBaseCode=LD  InternalSimscapePortConfiguration="{\"Bottom\":[],\"Left\":[{\"id\":\"S\",\"label\":\"S\",\"type\":\"foundation.mechanical.translational.translational\"},{\"id\":\"R\",\"label\":\"R\",\"type\":\"foundation.mechanical.rotational.rotational\"}],\"Right\":[{\"id\":\"X\",\"label\":\"X\",\"type\":\"output\"},{\"id\":\"H\",\"label\":\"H\",\"type\":\"foundation.mechanical.rotational.rotational\"}],\"Top\":[]}"
  HighPawl : sdl_lib/Clutches/Dog Clutch  thermal_port=simscape.enum.thermaleffects.omit  model=1  max_torque=1000 N*m  temperature_TLU=[280.0, 300.0, 320.0] K  max_torque_vector=[1000.0, 1050.0, 1000.0] N*m  interp_method=1  extrap_method=1  radius=10 mm  n_teeth=6  clutch_backlash=10 deg  clutch_stiffness=1e+7 N*m/rad  clutch_damping=100 N*m/(rad/s)  shift_linkage=sdl.enum.shift_linkage.conserving  tooth_height=3 mm  ring_hub_gap=1 mm  back_stop=1  transl_stiffness=1e+6 N/m  transl_damping=1000 N/(m/s)  visc_fric_transl=100 N/(m/s)  fric_coeff=0.05  direction=3-2*(1)  engagement_velocity=inf rpm  engagement_overlap=1 mm  initial_state_engaged=0  init_pos=0 mm  init_rel_angle=0 deg  thermal_mass=25 kJ/K  T_init=300 K
      settings: SourceProductBaseCode=LD  InternalSimscapePortConfiguration="{\"Bottom\":[],\"Left\":[{\"id\":\"S\",\"label\":\"S\",\"type\":\"foundation.mechanical.translational.translational\"},{\"id\":\"R\",\"label\":\"R\",\"type\":\"foundation.mechanical.rotational.rotational\"}],\"Right\":[{\"id\":\"X\",\"label\":\"X\",\"type\":\"output\"},{\"id\":\"H\",\"label\":\"H\",\"type\":\"foundation.mechanical.rotational.rotational\"}],\"Top\":[]}"
  Hub Inertia : fl_lib/Mechanical/Rotational Elements/Inertia  inertia=0.0005 kg*m^2  num_ports=foundation.enum.numPorts2.one  w_specify=on  w_priority=High  w=0 rad/s  w_nominal_specify=off  w_nominal_unit=rad/s  w_nominal_value=1  t_specify=off  t_priority=High  t=0 N*m  t_nominal_specify=off  t_nominal_unit=N*m  t_nominal_value=1
  Low Actuator : clutch_lib/Clutch Actuator  SystemSampleTime=-1  VariantActivationTime=update diagram  Latency=0  AutoFrameSizeCalculation=off
  LowClutch : sdl_lib/Clutches/Dog Clutch  thermal_port=simscape.enum.thermaleffects.omit  model=1  max_torque=1000 N*m  temperature_TLU=[280.0, 300.0, 320.0] K  max_torque_vector=[1000.0, 1050.0, 1000.0] N*m  interp_method=1  extrap_method=1  radius=10 mm  n_teeth=6  clutch_backlash=10 deg  clutch_stiffness=1e+7 N*m/rad  clutch_damping=100 N*m/(rad/s)  shift_linkage=sdl.enum.shift_linkage.conserving  tooth_height=3 mm  ring_hub_gap=1 mm  back_stop=1  transl_stiffness=1e+6 N/m  transl_damping=1000 N/(m/s)  visc_fric_transl=100 N/(m/s)  fric_coeff=0.05  direction=3-2*(1)  engagement_velocity=inf rpm  engagement_overlap=1.5 mm  initial_state_engaged=1  init_pos=3 mm  init_rel_angle=0 deg  thermal_mass=25 kJ/K  T_init=300 K
      settings: SourceProductBaseCode=LD  InternalSimscapePortConfiguration="{\"Bottom\":[],\"Left\":[{\"id\":\"S\",\"label\":\"S\",\"type\":\"foundation.mechanical.translational.translational\"},{\"id\":\"R\",\"label\":\"R\",\"type\":\"foundation.mechanical.rotational.rotational\"}],\"Right\":[{\"id\":\"X\",\"label\":\"X\",\"type\":\"output\"},{\"id\":\"H\",\"label\":\"H\",\"type\":\"foundation.mechanical.rotational.rotational\"}],\"Top\":[]}"
  LowPawl : sdl_lib/Clutches/Dog Clutch  thermal_port=simscape.enum.thermaleffects.omit  model=1  max_torque=1000 N*m  temperature_TLU=[280.0, 300.0, 320.0] K  max_torque_vector=[1000.0, 1050.0, 1000.0] N*m  interp_method=1  extrap_method=1  radius=10 mm  n_teeth=6  clutch_backlash=10 deg  clutch_stiffness=1e+7 N*m/rad  clutch_damping=100 N*m/(rad/s)  shift_linkage=sdl.enum.shift_linkage.conserving  tooth_height=3 mm  ring_hub_gap=1 mm  back_stop=1  transl_stiffness=1e+6 N/m  transl_damping=1000 N/(m/s)  visc_fric_transl=100 N/(m/s)  fric_coeff=0.05  direction=3-2*(1)  engagement_velocity=inf rpm  engagement_overlap=1.5 mm  initial_state_engaged=1  init_pos=3 mm  init_rel_angle=0 deg  thermal_mass=25 kJ/K  T_init=300 K
      settings: SourceProductBaseCode=LD  InternalSimscapePortConfiguration="{\"Bottom\":[],\"Left\":[{\"id\":\"S\",\"label\":\"S\",\"type\":\"foundation.mechanical.translational.translational\"},{\"id\":\"R\",\"label\":\"R\",\"type\":\"foundation.mechanical.rotational.rotational\"}],\"Right\":[{\"id\":\"X\",\"label\":\"X\",\"type\":\"output\"},{\"id\":\"H\",\"label\":\"H\",\"type\":\"foundation.mechanical.rotational.rotational\"}],\"Top\":[]}"
  Mechanical Rotational Reference : fl_lib/Mechanical/Rotational Elements/Mechanical Rotational Reference
  Mid Actuator : clutch_lib/Clutch Actuator  SystemSampleTime=-1  VariantActivationTime=update diagram  Latency=0  AutoFrameSizeCalculation=off
  MidClutch : sdl_lib/Clutches/Dog Clutch  thermal_port=simscape.enum.thermaleffects.omit  model=1  max_torque=1000 N*m  temperature_TLU=[280.0, 300.0, 320.0] K  max_torque_vector=[1000.0, 1050.0, 1000.0] N*m  interp_method=1  extrap_method=1  radius=10 mm  n_teeth=6  clutch_backlash=10 deg  clutch_stiffness=1e+7 N*m/rad  clutch_damping=100 N*m/(rad/s)  shift_linkage=sdl.enum.shift_linkage.conserving  tooth_height=3 mm  ring_hub_gap=1 mm  back_stop=1  transl_stiffness=1e+6 N/m  transl_damping=1000 N/(m/s)  visc_fric_transl=100 N/(m/s)  fric_coeff=0.05  direction=3-2*(1)  engagement_velocity=inf rpm  engagement_overlap=1.5 mm  initial_state_engaged=0  init_pos=0 mm  init_rel_angle=0 deg  thermal_mass=25 kJ/K  T_init=300 K
      settings: SourceProductBaseCode=LD  InternalSimscapePortConfiguration="{\"Bottom\":[],\"Left\":[{\"id\":\"S\",\"label\":\"S\",\"type\":\"foundation.mechanical.translational.translational\"},{\"id\":\"R\",\"label\":\"R\",\"type\":\"foundation.mechanical.rotational.rotational\"}],\"Right\":[{\"id\":\"X\",\"label\":\"X\",\"type\":\"output\"},{\"id\":\"H\",\"label\":\"H\",\"type\":\"foundation.mechanical.rotational.rotational\"}],\"Top\":[]}"
  MidPawl : sdl_lib/Clutches/Dog Clutch  thermal_port=simscape.enum.thermaleffects.omit  model=1  max_torque=1000 N*m  temperature_TLU=[280.0, 300.0, 320.0] K  max_torque_vector=[1000.0, 1050.0, 1000.0] N*m  interp_method=1  extrap_method=1  radius=10 mm  n_teeth=6  clutch_backlash=10 deg  clutch_stiffness=1e+7 N*m/rad  clutch_damping=100 N*m/(rad/s)  shift_linkage=sdl.enum.shift_linkage.conserving  tooth_height=3 mm  ring_hub_gap=1 mm  back_stop=1  transl_stiffness=1e+6 N/m  transl_damping=1000 N/(m/s)  visc_fric_transl=100 N/(m/s)  fric_coeff=0.05  direction=3-2*(1)  engagement_velocity=inf rpm  engagement_overlap=1.5 mm  initial_state_engaged=0  init_pos=0 mm  init_rel_angle=0 deg  thermal_mass=25 kJ/K  T_init=300 K
      settings: SourceProductBaseCode=LD  InternalSimscapePortConfiguration="{\"Bottom\":[],\"Left\":[{\"id\":\"S\",\"label\":\"S\",\"type\":\"foundation.mechanical.translational.translational\"},{\"id\":\"R\",\"label\":\"R\",\"type\":\"foundation.mechanical.rotational.rotational\"}],\"Right\":[{\"id\":\"X\",\"label\":\"X\",\"type\":\"output\"},{\"id\":\"H\",\"label\":\"H\",\"type\":\"foundation.mechanical.rotational.rotational\"}],\"Top\":[]}"
  PS-Simulink Converter{,1..5} (6 alike) : nesl_utility/PS-Simulink Converter  PhysicalDomain=network_engine_domain  SubClassName=ps_output  LeftPortType=input  RightPortType=output  PseudoPeriodic=off  Frequencies=[]  Unit=mm  AffineConversion=off
  Planetary Gear : sdl_lib/Gears/Planetary Gear  rs_ratio=2  friction_model=1  mu_visc=[ 0 0 ] N*m/(rad/s)  efficiency=[ 0.96 0.98 ]  temperature_TLU=[ 280 300 320 ] K  efficiency_sp_TLU=[ 0.95 0.9 0.85 ]  efficiency_rp_TLU=[ 0.95 0.9 0.85 ]  pwr_thr=[ 0.001 0.001 ] W  thermal_mass=50 J/K  T_init=300 K  model_inertia=0  planet_inertia=0.001 kg*m^2
      settings: SourceProductBaseCode=LD
  Ring Inertia : fl_lib/Mechanical/Rotational Elements/Inertia  inertia=0.0005 kg*m^2  num_ports=foundation.enum.numPorts2.one  w_specify=on  w_priority=High  w=0 rad/s  w_nominal_specify=off  w_nominal_unit=rad/s  w_nominal_value=1  t_specify=off  t_priority=High  t=0 N*m  t_nominal_specify=off  t_nominal_unit=N*m  t_nominal_value=1
  Terminator : Terminator
  Terminator1 : Terminator
  Terminator2 : Terminator
  A : PMIOPort  Side=Left
  H : PMIOPort  Port=2  Side=Right
  wires:
  Cmd/1 -> Compare To Constant2/1, Compare To Constant1/1, Compare To Constant/1
  Compare To Constant1/1 -> [High]
  [Low] -> GearSelect/1
  [Mid] -> GearSelect/2
  [High] -> GearSelect/3
  Compare To Constant2/1 -> [Low]
  Compare To Constant/1 -> [Mid]
  [Mid] -> Mid Actuator/1
  PS-Simulink Converter/1 -> [InMid]
  PS-Simulink Converter1/1 -> Terminator/1
  [InMid] -> ClutchPos/2
  [Low] -> Low Actuator/1
  PS-Simulink Converter2/1 -> [InLow]
  PS-Simulink Converter3/1 -> Terminator1/1
  [InLow] -> ClutchPos/1
  [High] -> High Actuator/1
  PS-Simulink Converter4/1 -> [InHigh]
  [InHigh] -> ClutchPos/3
  PS-Simulink Converter5/1 -> Terminator2/1
  connections:
  MidPawl/LConn1 -- MidClutch/LConn1 -- Mid Actuator/RConn1
  A/RConn1 -- MidClutch/LConn2 -- LowClutch/LConn2 -- HighClutch/LConn2
  MidPawl/RConn2 -- H/RConn1 -- HighPawl/RConn2 -- LowPawl/RConn2
  MidClutch/RConn1 -- PS-Simulink Converter/LConn1
  MidPawl/RConn1 -- PS-Simulink Converter1/LConn1
  LowClutch/LConn1 -- LowPawl/LConn1 -- Low Actuator/RConn1
  MidPawl/LConn2 -- MidClutch/RConn2 -- Hub Inertia/LConn1
  LowClutch/RConn2 -- Ring Inertia/LConn1 -- HighPawl/LConn2 -- Planetary Gear/RConn1
  Carrier Inertia/LConn1 -- Planetary Gear/LConn1 -- LowPawl/LConn2 -- HighClutch/RConn2
  PS-Simulink Converter2/LConn1 -- LowClutch/RConn1
  PS-Simulink Converter3/LConn1 -- LowPawl/RConn1
  HighClutch/RConn1 -- PS-Simulink Converter4/LConn1
  Mechanical Rotational Reference/LConn1 -- Planetary Gear/RConn2
  HighPawl/LConn1 -- HighClutch/LConn1 -- High Actuator/RConn1
  PS-Simulink Converter5/LConn1 -- HighPawl/RConn1

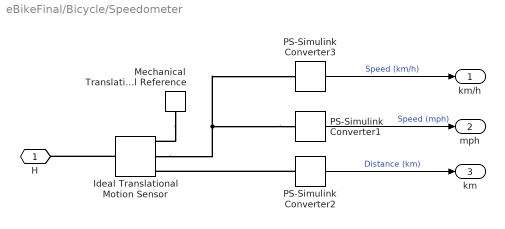
== system eBikeFinal/Bicycle/Speedometer ==
  Ideal Translational Motion Sensor : fl_lib/Mechanical/Mechanical Sensors/Ideal Translational Motion Sensor  offset=0 m
  Mechanical Translational Reference : fl_lib/Mechanical/Translational Elements/Mechanical Translational Reference
  PS-Simulink Converter1 : nesl_utility/PS-Simulink Converter  PhysicalDomain=network_engine_domain  SubClassName=ps_output  LeftPortType=input  RightPortType=output  PseudoPeriodic=off  Frequencies=[]  Unit=mi/hr  AffineConversion=off
  PS-Simulink Converter2 : nesl_utility/PS-Simulink Converter  PhysicalDomain=network_engine_domain  SubClassName=ps_output  LeftPortType=input  RightPortType=output  PseudoPeriodic=off  Frequencies=[]  Unit=km  AffineConversion=off
  PS-Simulink Converter3 : nesl_utility/PS-Simulink Converter  PhysicalDomain=network_engine_domain  SubClassName=ps_output  LeftPortType=input  RightPortType=output  PseudoPeriodic=off  Frequencies=[]  Unit=km/hr  AffineConversion=off
  H : PMIOPort  Side=Left
  km/h : Outport  VectorParamsAs1DForOutWhenUnconnected=off
  mph : Outport  Port=2  VectorParamsAs1DForOutWhenUnconnected=off
  km : Outport  Port=3  VectorParamsAs1DForOutWhenUnconnected=off
  wires:
  PS-Simulink Converter3/1 -> km/h/1  "Speed (km/h)"
  PS-Simulink Converter1/1 -> mph/1  "Speed (mph)"
  PS-Simulink Converter2/1 -> km/1  "Distance (km)"
  connections:
  PS-Simulink Converter1/LConn1 -- PS-Simulink Converter3/LConn1 -- Ideal Translational Motion Sensor/RConn2
  PS-Simulink Converter2/LConn1 -- Ideal Translational Motion Sensor/RConn3
  Ideal Translational Motion Sensor/LConn1 -- H/RConn1
  Mechanical Translational Reference/LConn1 -- Ideal Translational Motion Sensor/RConn1
